simulink model "assignment_2_1"  (R2023b)
settings: Solver=ode1  StartTime=0.0  StopTime=30  FixedStep=0.001  RelTol=1e-3
undefined symbols (not defined in the file): den, num
settings Model: Creator=bengo  LastModifiedBy=bengo

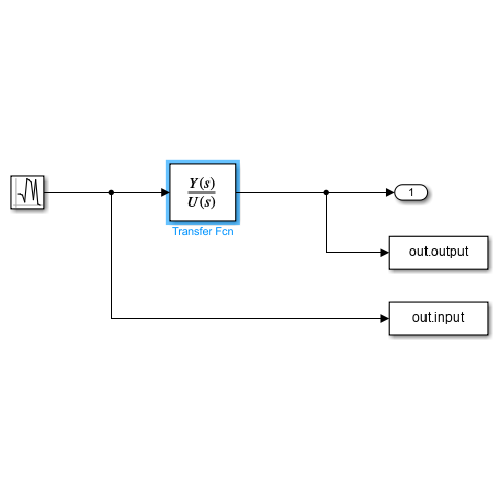
[thumbnail: Simulink's stored preview of the top-level diagram]
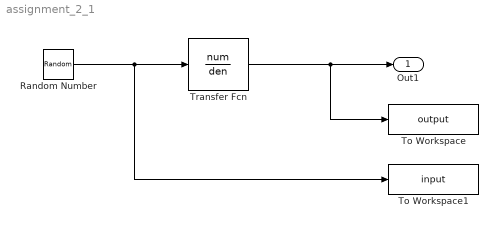
== system assignment_2_1 ==
  Random Number : RandomNumber  SampleTime=0.001
  To Workspace : ToWorkspace  VariableName=output  SaveFormat=Timeseries  SampleTime=-1
  To Workspace1 : ToWorkspace  VariableName=input  SaveFormat=Timeseries  SampleTime=-1
  Transfer Fcn : TransferFcn  Numerator=num  Denominator=den
  Out1 : Outport
  wires:
  Random Number/1 -> To Workspace1/1, Transfer Fcn/1
  Transfer Fcn/1 -> To Workspace/1, Out1/1
